simulink model "mseCaseMuxOfFour"  (R2023b)
settings: Solver=VariableStepAuto  StartTime=0.0  StopTime=10.0  RelTol=1e-3
settings Model: Creator=DarianMuresan  LastModifiedBy=DarianMuresan

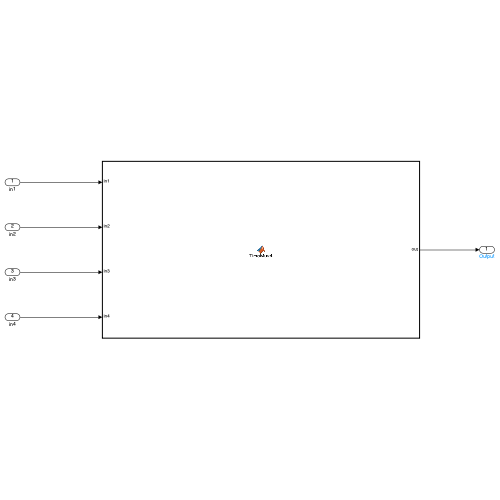
[thumbnail: Simulink's stored preview of the top-level diagram]
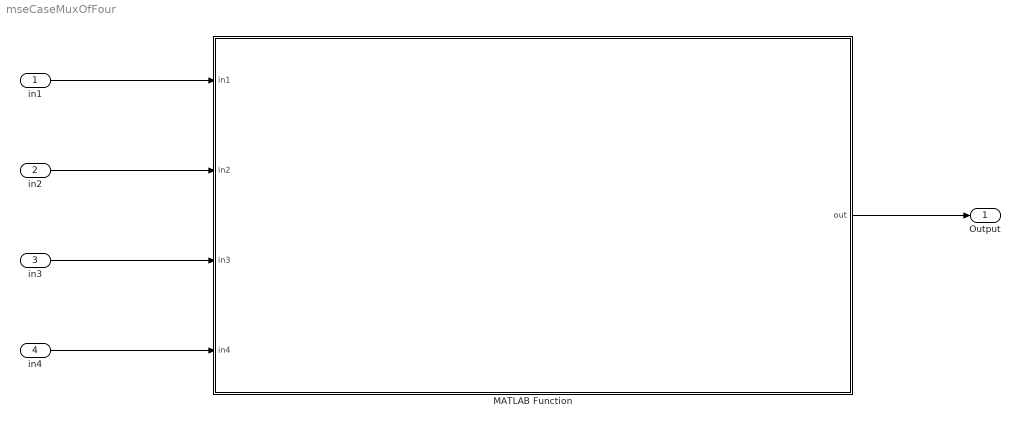
== system mseCaseMuxOfFour ==
  in1 : Inport
  in2 : Inport  Port=2
  in3 : Inport  Port=3
  in4 : Inport  Port=4
  MATLAB Function : MATLAB Function  TreatAsAtomicUnit=on
  Output : Outport
  wires:
  in4/1 -> MATLAB Function/4(in4)
  in3/1 -> MATLAB Function/3(in3)
  in2/1 -> MATLAB Function/2(in2)
  in1/1 -> MATLAB Function/1(in1)
  MATLAB Function/1(out) -> Output/1

== matlab function mseCaseMuxOfFour/MATLAB Function ==
  data: in1 input; out output; in2 input; in3 input; in4 input
function out = mseCaseMuxOfFour(in1,in2,in3,in4)

% Method to mux 4 inputs into one of 4 possible outputs based on
% the first non-negative input.  To be paired with CaseSplitOfFour.
%
% Written by: Darian Muresan
% Last Modified: 10/10/2024

if nargin<2
    in2=-1;
    in3=-1;
    in4=-1;
elseif nargin<3
    in3=-1;
    in4=-1;
elseif nargin<4
    in4=-1;
end

if in1>=0
    out = in1;
elseif in2>=0
    out = in2;
elseif in3>=0
    out = in3;
elseif in4>=0
    out = in4;
else
    out = -1;
end
